simulink library "TQR_lib"  (Simulink 7.5)
settings: Solver=ode45  StartTime=0.0  StopTime=10.0  RelTol=1e-3
values from neighbouring files (symbols this model uses):
  p1_ACPI_PICFilDen1_na = Simulink.Parameter    [TQR_par.m]
  p1_ACPI_PICFilDen2_na = Simulink.Parameter    [TQR_par.m]
  p1_ACPI_PICFilDen3_na = Simulink.Parameter    [TQR_par.m]
  p1_ACPI_PICFilNum1_na = Simulink.Parameter    [TQR_par.m]
  p1_ACPI_PICFilNum2_na = Simulink.Parameter    [TQR_par.m]
  p1_ACPI_PICFilNum3_na = Simulink.Parameter    [TQR_par.m]
  pTQR_bar_BrkPOvrdRecoverThd_C = Simulink.Parameter    [TQR_par.m]
  pTQR_bar_BrkPOvrdVal_C = Simulink.Parameter    [TQR_par.m]
  pTQR_bar_ECrpTrqStrtPres_C = Simulink.Parameter    [TQR_par.m]
  pTQR_bar_MasterCylPres_CUR = Simulink.Parameter    [TQR_par.m]
  pTQR_bool_AccPedOvrdDsbl_C = Simulink.Parameter    [TQR_par.m]
  pTQR_bool_BrkPOvrdDsbl_C = Simulink.Parameter    [TQR_par.m]
  pTQR_bool_BrkRecupSrcSelSwt_C = Simulink.Parameter    [TQR_par.m]
  pTQR_bool_PICTqEna_C = Simulink.Parameter    [TQR_par.m]
  pTQR_bool_RecupEna_C = Simulink.Parameter    [TQR_par.m]
  pTQR_kmph_MaxVehSpd_C = Simulink.Parameter    [TQR_par.m]
  pTQR_kmph_MinVehSpd_C = Simulink.Parameter    [TQR_par.m]
  pTQR_kmph_VehSpd_TAB = Simulink.Parameter    [TQR_par.m]
  pTQR_kmph_VehSpdMaxDriving_TAB = Simulink.Parameter    [TQR_par.m]
  pTQR_kmph_VehSpdMaxReverse_TAB = Simulink.Parameter    [TQR_par.m]
  pTQR_kmph_VehSpdRednHi_CUR = Simulink.Parameter    [TQR_par.m]
  pTQR_kmph_VehSpdRednLo_CUR = Simulink.Parameter    [TQR_par.m]
  pTQR_Nm_ACCDelyOutTrq_C = Simulink.Parameter    [TQR_par.m]
  pTQR_Nm_ACCOutTrqLo_C = Simulink.Parameter    [TQR_par.m]
  pTQR_Nm_ACCOutTrqUp_C = Simulink.Parameter    [TQR_par.m]
  pTQR_Nm_BrkECrpTrq_TAB = Simulink.Parameter    [TQR_par.m]
  pTQR_Nm_MaxRecupTq_C = Simulink.Parameter    [TQR_par.m]
  pTQR_Nm_MotCtlrMaxTqLim_C = Simulink.Parameter    [TQR_par.m]
  pTQR_Nm_MotCtlrMinTqLim_C = Simulink.Parameter    [TQR_par.m]
  pTQR_Nm_PreloadTrq_C = Simulink.Parameter    [TQR_par.m]
  pTQR_Nm_PRNDLoTbl_MAP = Simulink.Parameter    [TQR_par.m]
  pTQR_Nm_RecupLoTbl_MAP = Simulink.Parameter    [TQR_par.m]
  pTQR_Nm_REDEVPRNDLoTbl_MAP = Simulink.Parameter    [TQR_par.m]
  pTQR_Nm_TqLimnUpprLim_C = Simulink.Parameter    [TQR_par.m]
  pTQR_Nmps_AccPedValLowrRateLim_CUR = Simulink.Parameter    [TQR_par.m]
  pTQR_Nmps_AccPedValUpprRateLim_CUR = Simulink.Parameter    [TQR_par.m]
  pTQR_Nmps_CrsCtlLowrRateLim_C = Simulink.Parameter    [TQR_par.m]
  pTQR_Nmps_CrsCtlUpprRateLim_C = Simulink.Parameter    [TQR_par.m]
  pTQR_Nmps_FltLowrRateLim_C = Simulink.Parameter    [TQR_par.m]
  pTQR_Nmps_FltUpprRateLim_C = Simulink.Parameter    [TQR_par.m]
  pTQR_Nmps_LowrRateLimLoTbl_TAB = Simulink.Parameter    [TQR_par.m]
  pTQR_Nmps_UpprRateLimLoTbl_TAB = Simulink.Parameter    [TQR_par.m]
  pTQR_pct_AccPedAcvThd_C = Simulink.Parameter    [TQR_par.m]
  pTQR_pct_AccPedOvrdRecThd_C = Simulink.Parameter    [TQR_par.m]
  pTQR_pct_AccPedOvrdVal_C = Simulink.Parameter    [TQR_par.m]
  pTQR_pct_AccPedThCC_C = Simulink.Parameter    [TQR_par.m]
  pTQR_pct_BrkPOvrdAccPedValThd_C = Simulink.Parameter    [TQR_par.m]
  pTQR_pct_PICAccPedValThd_C = Simulink.Parameter    [TQR_par.m]
  pTQR_r_BrkDwnFilterFac_C = Simulink.Parameter    [TQR_par.m]
  pTQR_r_BrkUpFilterFac_C = Simulink.Parameter    [TQR_par.m]
  pTQR_r_BrkWeightDsbl_C = Simulink.Parameter    [TQR_par.m]
  pTQR_r_BrkWeightFac_C = Simulink.Parameter    [TQR_par.m]
  pTQR_r_ECrpShfFilterFac_C = Simulink.Parameter    [TQR_par.m]
  pTQR_r_PICFilDen1_C = Simulink.Parameter    [TQR_par.m]
  pTQR_r_PICFilDen2_C = Simulink.Parameter    [TQR_par.m]
  pTQR_r_PICFilDen3_C = Simulink.Parameter    [TQR_par.m]
  pTQR_r_PICFilNum1_C = Simulink.Parameter    [TQR_par.m]
  pTQR_r_PICFilNum2_C = Simulink.Parameter    [TQR_par.m]
  pTQR_r_PICFilNum3_C = Simulink.Parameter    [TQR_par.m]
  pTQR_r_PreloadFilterFac_C = Simulink.Parameter    [TQR_par.m]
  pTQR_r_TrqDwnFilterFac_MAP = [ ... (first row only)    [TQR_par.m]
  pTQR_r_TrqUppFilterFac_MAP = [ ... (first row only)    [TQR_par.m]
  pTQR_r_VehSpdFilterFac_CUR = Simulink.Parameter    [TQR_par.m]
  pTQR_ratio_AccPedOvrdLoRate_C = Simulink.Parameter    [TQR_par.m]
  pTQR_ratio_AccPedOvrdUpRate_C = Simulink.Parameter    [TQR_par.m]
  pTQR_ratio_AccPedTqLimUpRate_C = Simulink.Parameter    [TQR_par.m]
  pTQR_ratio_BrkOvrAccPedGrdTh_C = Simulink.Parameter    [TQR_par.m]
  pTQR_ratio_BrkPOvrdLoRate_C = Simulink.Parameter    [TQR_par.m]
  pTQR_ratio_BrkPOvrdUpRate_C = Simulink.Parameter    [TQR_par.m]
  pTQR_ratio_PerfIdxGain_C = Simulink.Parameter    [TQR_par.m]
  pTQR_rpm_VehMoveSpdThrsh_C = Simulink.Parameter    [TQR_par.m]
  pTQR_rpm_VehStdStlSpdThrsh_C = Simulink.Parameter    [TQR_par.m]
  pTQR_s_AccPedActDly_C = Simulink.Parameter    [TQR_par.m]
  pTQR_s_ShfPreloadTrqTmrDly_C = Simulink.Parameter    [TQR_par.m]
  pTQR_s_ShfTrqTmrDly_C = Simulink.Parameter    [TQR_par.m]
  pTQR_s_SmplCyc_C = Simulink.Parameter    [TQR_par.m]
  pTQR_s_VehStdStlDly_C = Simulink.Parameter    [TQR_par.m]
undefined symbols (not defined in the file or in its folder): CrsCtlStsTyp, DiscIntNeverNeededParam, p_single_Minus_M, p_single_Zero_M, ShiftLvrPosnTyp
libraries: BaseOperationLib_Browser x214, simulink x11, PES_CZ_FAW x2, simulink_extras x2, A0EV_Lib1 x1
(part 2 of 2)

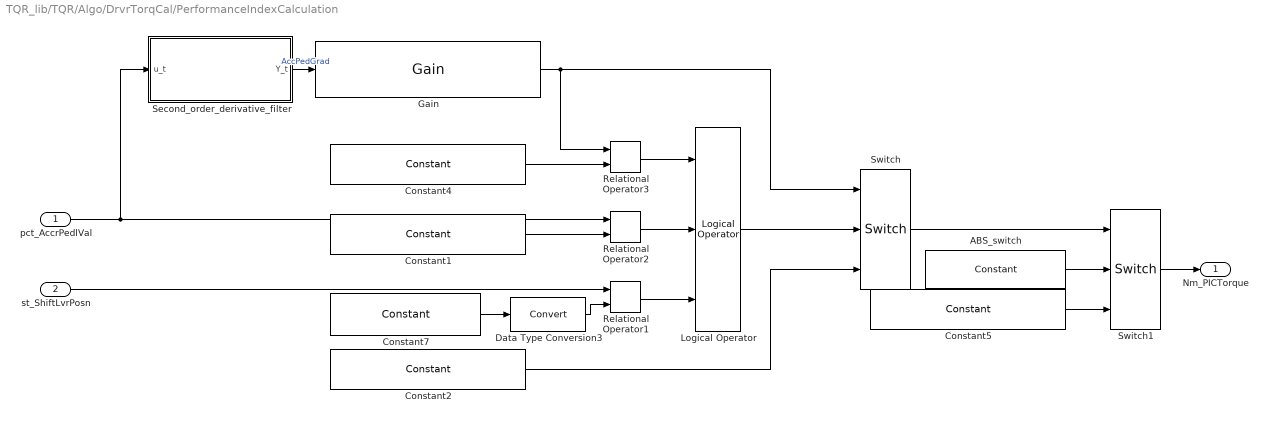
== system TQR_lib/TQR/Algo/DrvrTorqCal/PerformanceIndexCalculation ==
  pct_AccrPedlVal : Inport
  st_ShiftLvrPosn : Inport  Port=2
  ABS_switch : BaseOperationLib_Browser/Sources&Sinks/Constant  Value=pTQR_bool_PICTqEna_C  OutMin=[]  OutMax=[]  OutDataTypeMode=boolean  OutDataType=fixdt(1, 16)  ConRadixGroup=Use specified scaling  OutScaling=2^0  OutDataTypeStr=boolean
  Constant1 : BaseOperationLib_Browser/Sources&Sinks/Constant  Value=pTQR_pct_PICAccPedValThd_C  OutMin=[]  OutMax=[]  OutDataType=fixdt(1, 16)  ConRadixGroup=Use specified scaling  OutScaling=2^0  OutDataTypeStr=Inherit: Inherit from 'Constant value'
  Constant2 : BaseOperationLib_Browser/Sources&Sinks/Constant  Value=p_single_Zero_M  OutMin=[]  OutMax=[]  OutDataType=fixdt(1, 16)  ConRadixGroup=Use specified scaling  OutScaling=2^0  OutDataTypeStr=Inherit: Inherit from 'Constant value'
  Constant4 : BaseOperationLib_Browser/Sources&Sinks/Constant  Value=p_single_Zero_M  OutMin=[]  OutMax=[]  OutDataType=fixdt(1, 16)  ConRadixGroup=Use specified scaling  OutScaling=2^0  OutDataTypeStr=Inherit: Inherit from 'Constant value'
  Constant5 : BaseOperationLib_Browser/Sources&Sinks/Constant  Value=p_single_Zero_M  OutMin=[]  OutMax=[]  OutDataType=fixdt(1, 16)  ConRadixGroup=Use specified scaling  OutScaling=2^0  OutDataTypeStr=Inherit: Inherit from 'Constant value'
  Constant7 : BaseOperationLib_Browser/Sources&Sinks/Constant  Value=ShiftLvrPosnTyp.SHL_D  OutMin=[]  OutMax=[]  OutDataType=fixdt(1, 16)  ConRadixGroup=Use specified scaling  OutScaling=2^0  OutDataTypeStr=Inherit: Inherit from 'Constant value'
  Data Type Conversion3 : DataTypeConversion  OutDataType=fixdt(1, 16)  OutScaling=2^0
  Gain : BaseOperationLib_Browser/Math Operations Changed/Gain  Gain=pTQR_ratio_PerfIdxGain_C  Multiplication=Element-wise(K.*u)  ParamMin=[]  ParamMax=[]  ParameterDataType=fixdt(1, 16)  ParameterScalingMode=Best Precision: Matrix-wise  ParameterScaling=2^0  OutMin=[]  OutMax=[]  OutDataType=fixdt(1, 16)  OutScaling=2^0  OutDataTypeStr=Inherit: Inherit via back propagation
  Logical Operator : BaseOperationLib_Browser/Logic Operations Changed/Logical Operator  Operator=AND  Inputs=3  AllPortsSameDT=off  OutDataTypeMode=boolean  LogicDataType=PDT_Bool  OutDataTypeStr=boolean
  Relational Operator1 : BaseOperationLib_Browser/Logic Operations Changed/Relational Operator  Operator===  LogicOutDataTypeMode=boolean  LogicDataType=PDT_Bool  OutDataTypeStr=boolean
  Relational Operator2 : BaseOperationLib_Browser/Logic Operations Changed/Relational Operator  Operator=>  LogicOutDataTypeMode=boolean  LogicDataType=PDT_Bool  OutDataTypeStr=boolean
  Relational Operator3 : BaseOperationLib_Browser/Logic Operations Changed/Relational Operator  Operator=>  LogicOutDataTypeMode=boolean  LogicDataType=PDT_Bool  OutDataTypeStr=boolean
  Second_order_derivative_filter : Subsystem
  Switch : BaseOperationLib_Browser/Signal Routing Changed/Switch  Criteria=u2 ~= 0  Threshold=0  OutMin=[]  OutMax=[]  OutDataType=fixdt(1,16,0)  OutScaling=[]
  Switch1 : BaseOperationLib_Browser/Signal Routing Changed/Switch  Criteria=u2 ~= 0  Threshold=0  OutMin=[]  OutMax=[]  OutDataType=fixdt(1,16,0)  OutScaling=[]
  Nm_PICTorque : Outport
  wires:
  Gain/1 -> Switch/1, Relational Operator3/1
  Constant2/1 -> Switch/3
  Logical Operator/1 -> Switch/2
  pct_AccrPedlVal/1 -> Relational Operator2/1, Second_order_derivative_filter/1(u_t)
  Constant1/1 -> Relational Operator2/2
  Second_order_derivative_filter/1(Y_t) -> Gain/1  "AccPedGrad"
  Relational Operator3/1 -> Logical Operator/1
  Constant4/1 -> Relational Operator3/2
  Relational Operator2/1 -> Logical Operator/2
  Switch/1 -> Switch1/1
  Constant5/1 -> Switch1/3
  ABS_switch/1 -> Switch1/2
  Switch1/1 -> Nm_PICTorque/1
  Data Type Conversion3/1 -> Relational Operator1/2
  Constant7/1 -> Data Type Conversion3/1
  Relational Operator1/1 -> Logical Operator/3
  st_ShiftLvrPosn/1 -> Relational Operator1/1

== system TQR_lib/TQR/Algo/DrvrTorqCal/SlpVehLgtSpdTrans ==
  kmph_VehLgtSpd : Inport
  st_ShiftLvrPosn : Inport  Port=2
  Constant1 : BaseOperationLib_Browser/Sources&Sinks/Constant  Value=pTQR_kmph_MaxVehSpd_C  OutMin=[]  OutMax=[]  OutDataType=fixdt(1, 16)  ConRadixGroup=Use specified scaling  OutScaling=2^0  OutDataTypeStr=Inherit: Inherit from 'Constant value'
  Constant3 : BaseOperationLib_Browser/Sources&Sinks/Constant  Value=pTQR_kmph_MinVehSpd_C  OutMin=[]  OutMax=[]  OutDataType=fixdt(1, 16)  ConRadixGroup=Use specified scaling  OutScaling=2^0  OutDataTypeStr=Inherit: Inherit from 'Constant value'
  Constant7 : BaseOperationLib_Browser/Sources&Sinks/Constant  Value=ShiftLvrPosnTyp.SHL_R  OutMin=[]  OutMax=[]  OutDataType=fixdt(1, 16)  ConRadixGroup=Use specified scaling  OutScaling=2^0  OutDataTypeStr=Inherit: Inherit from 'Constant value'
  Data Type Conversion3 : DataTypeConversion  OutDataType=fixdt(1, 16)  OutScaling=2^0
  ECrpVehSpdFilter : Subsystem
  Gain : BaseOperationLib_Browser/Math Operations Changed/Gain  Gain=p_single_Minus_M  Multiplication=Element-wise(K.*u)  ParamMin=[]  ParamMax=[]  ParameterDataType=fixdt(1, 16)  ParameterScalingMode=Best Precision: Matrix-wise  ParameterScaling=2^0  ParamDataTypeStr=Inherit: Inherit from 'Gain'  OutMin=[]  OutMax=[]  OutDataType=fixdt(1, 16)  OutScaling=2^0  SaturateOnIntegerOverflow=on
  Relational Operator1 : BaseOperationLib_Browser/Logic Operations Changed/Relational Operator  Operator===  LogicOutDataTypeMode=boolean  LogicDataType=PDT_Bool  OutDataTypeStr=boolean
  Saturation Dynamic : BaseOperationLib_Browser/Discontinuities Unchanged/Saturation Dynamic  SystemSampleTime=-1  OutMin=[]  OutMax=[]  OutDataTypeStr=Inherit: Same as second input  OutDataType=fixdt(1, 16)  OutScaling=2^-10  DoSatur=off
  Switch2 : BaseOperationLib_Browser/Signal Routing Changed/Switch  Criteria=u2 ~= 0  Threshold=0  OutMin=[]  OutMax=[]  OutDataType=fixdt(1,16,0)  OutScaling=[]
  kmph_SlpVehLgtSpdTrans : Outport
  wires:
  Data Type Conversion3/1 -> Relational Operator1/2
  Constant7/1 -> Data Type Conversion3/1
  Relational Operator1/1 -> Switch2/2
  kmph_VehLgtSpd/1 -> Switch2/3, Gain/1
  st_ShiftLvrPosn/1 -> Relational Operator1/1
  Constant3/1 -> Saturation Dynamic/3
  Constant1/1 -> Saturation Dynamic/1
  Switch2/1 -> Saturation Dynamic/2
  ECrpVehSpdFilter/1(kmph_VehSpdFilter) -> kmph_SlpVehLgtSpdTrans/1
  Saturation Dynamic/1 -> ECrpVehSpdFilter/1(kmph_VehSpd)
  Gain/1 -> Switch2/1

== system TQR_lib/TQR/Algo/DrvrTorqCal/velocity_limitation ==
  Nm_MotCtlrTqSp : Inport
  st_ShiftLvrPosn : Inport  Port=2
  kmph_VehLgtSpd : Inport  Port=3
  1-D Lookup Table_TQ_D : Lookup_n-D  NumberOfTableDimensions=1  BreakpointsForDimension1=pTQR_kmph_VehSpdMaxDriving_TAB  Table=[1 1 0 0]  RndMeth=Simplest  InputSameDT=on
  1-D Lookup Table_TQ_R : Lookup_n-D  NumberOfTableDimensions=1  BreakpointsForDimension1=pTQR_kmph_VehSpdMaxReverse_TAB  Table=[1 1 0 0]  RndMeth=Simplest  InputSameDT=on
  Abs : BaseOperationLib_Browser/Math Operations Changed/Abs  OutMax=[]  OutDataType=fixdt(1, 16)  OutScaling=2^0
  Compare To Zero : simulink/Logic and Bit Operations/Compare To Zero  SystemSampleTime=-1  relop=>  LogicOutDataTypeMode=uint8
  Constant : BaseOperationLib_Browser/Sources&Sinks/Constant  Value=ShiftLvrPosnTyp.SHL_R  OutMin=[]  OutMax=[]  OutDataTypeMode=Specify via dialog  OutDataType=Enum: ShiftLvrPosnTyp  ConRadixGroup=Best Precision: Vector-wise  OutScaling=[]  OutDataTypeStr=Enum: ShiftLvrPosnTyp
  Data Type Conversion1 : DataTypeConversion  OutDataType=fixdt(1, 16)  OutScaling=2^0
  Data Type Conversion2 : DataTypeConversion  OutDataTypeMode=Specify via dialog  OutDataType=Enum: ShiftLvrPosnTyp  OutDataTypeStr=Enum: ShiftLvrPosnTyp
  Product1 : BaseOperationLib_Browser/Math Operations Changed/Product  Inputs=2  Multiplication=Element-wise(.*)  OutMin=[]  OutMax=[]  OutDataType=fixdt(1,16,0)  OutScaling=[]  RndMeth=Zero
  Relational Operator : BaseOperationLib_Browser/Logic Operations Changed/Relational Operator  Operator===  LogicOutDataTypeMode=boolean  LogicDataType=PDT_Bool  OutDataTypeStr=boolean
  Switch : BaseOperationLib_Browser/Signal Routing Changed/Switch  Criteria=u2 ~= 0  Threshold=0  OutMin=[]  OutMax=[]  OutDataType=fixdt(1,16,0)  OutScaling=[]
  Switch1 : BaseOperationLib_Browser/Signal Routing Changed/Switch  Criteria=u2 ~= 0  Threshold=0  OutMin=[]  OutMax=[]  OutDataType=fixdt(1,16,0)  OutScaling=[]
  Nm_SpdLimitMotCtlrTqSp : Outport
  wires:
  Switch1/1 -> Data Type Conversion1/1
  Product1/1 -> Switch1/1
  Compare To Zero/1 -> Switch1/2
  Data Type Conversion2/1 -> Relational Operator/1
  Constant/1 -> Relational Operator/2
  Relational Operator/1 -> Switch/2
  1-D Lookup Table_TQ_D/1 -> Switch/3
  1-D Lookup Table_TQ_R/1 -> Switch/1
  Switch/1 -> Product1/1
  st_ShiftLvrPosn/1 -> Data Type Conversion2/1
  Nm_MotCtlrTqSp/1 -> Switch1/3, Product1/2, Compare To Zero/1
  kmph_VehLgtSpd/1 -> Abs/1
  Data Type Conversion1/1 -> Nm_SpdLimitMotCtlrTqSp/1
  Abs/1 -> 1-D Lookup Table_TQ_D/1, 1-D Lookup Table_TQ_R/1

== system TQR_lib/TQR/Algo/TorqArbitrition/DriveTorqArbitrition ==
  pct_AccrPedlVal : Inport
  Nm_CrsCtlTqSp : Inport  Port=2
  st_CrsCtlEna : Inport  Port=3
  Nm_TorqueRaw : Inport  Port=4
  Compare To Constant1 : BaseOperationLib_Browser/Logic Operations Changed/Compare To Constant  SystemSampleTime=-1  relop=>=  const=pTQR_pct_AccPedThCC_C
  Constant1 : BaseOperationLib_Browser/Sources&Sinks/Constant  Value=uint8(CrsCtlStsTyp.CCS_ACTIVE)  OutMin=[]  OutMax=[]  OutDataType=fixdt(1, 16)  ConRadixGroup=Use specified scaling  OutScaling=2^0  OutDataTypeStr=Inherit: Inherit from 'Constant value'
  Logical Operator : BaseOperationLib_Browser/Logic Operations Changed/Logical Operator  Operator=AND  Inputs=2  AllPortsSameDT=off  OutDataTypeMode=boolean  LogicDataType=PDT_Bool  OutDataTypeStr=boolean
  Logical Operator4 : BaseOperationLib_Browser/Logic Operations Changed/Logical Operator  Operator=NOT  Inputs=3  AllPortsSameDT=off  OutDataTypeMode=boolean  LogicDataType=PDT_Bool  OutDataTypeStr=boolean
  Logical Operator5 : BaseOperationLib_Browser/Logic Operations Changed/Logical Operator  Operator=OR  Inputs=2  AllPortsSameDT=off  OutDataTypeMode=boolean  LogicDataType=PDT_Bool  OutDataTypeStr=boolean
  MinMax : BaseOperationLib_Browser/Math Operations Changed/MinMax  Function=max  Inputs=2  OutMin=[]  OutMax=[]  OutDataType=fixdt(1, 16)  OutScaling=2^0
  Relational Operator : BaseOperationLib_Browser/Logic Operations Changed/Relational Operator  Operator=>=  LogicOutDataTypeMode=boolean  LogicDataType=PDT_Bool  OutDataTypeStr=boolean
  Relational Operator2 : BaseOperationLib_Browser/Logic Operations Changed/Relational Operator  Operator===  LogicOutDataTypeMode=boolean  LogicDataType=PDT_Bool  OutDataTypeStr=boolean
  Switch1 : BaseOperationLib_Browser/Signal Routing Changed/Switch  Criteria=u2 ~= 0  Threshold=0  OutMin=[]  OutMax=[]  OutDataType=fixdt(1,16,0)  OutScaling=[]
  Switch2 : BaseOperationLib_Browser/Signal Routing Changed/Switch  Criteria=u2 ~= 0  Threshold=0  OutMin=[]  OutMax=[]  OutDataType=fixdt(1,16,0)  OutScaling=[]
  Nm_DriveTorq : Outport
  bool_CrsCtlActive : Outport  Port=2
  wires:
  Constant1/1 -> Relational Operator2/1
  Switch2/1 -> Switch1/1
  MinMax/1 -> Switch2/1
  Compare To Constant1/1 -> Switch2/2, Logical Operator4/1
  Nm_TorqueRaw/1 -> MinMax/2, Switch1/3, Relational Operator/2
  Nm_CrsCtlTqSp/1 -> Switch2/3, MinMax/1, Relational Operator/1
  Relational Operator/1 -> Logical Operator5/2
  Logical Operator4/1 -> Logical Operator5/1
  Logical Operator5/1 -> Logical Operator/1
  Relational Operator2/1 -> Switch1/2, Logical Operator/2
  pct_AccrPedlVal/1 -> Compare To Constant1/1
  Switch1/1 -> Nm_DriveTorq/1
  st_CrsCtlEna/1 -> Relational Operator2/2
  Logical Operator/1 -> bool_CrsCtlActive/1

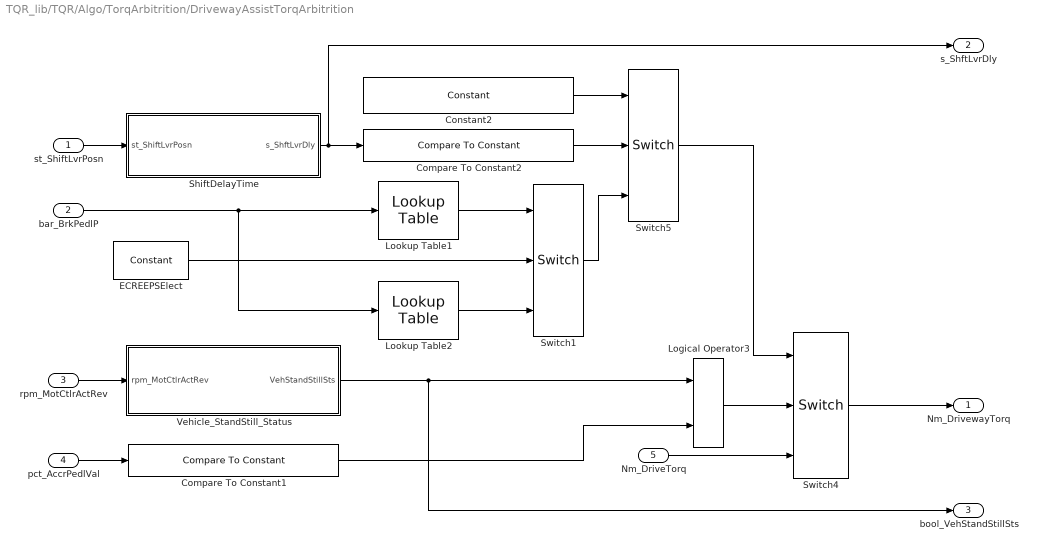
== system TQR_lib/TQR/Algo/TorqArbitrition/DrivewayAssistTorqArbitrition ==
  st_ShiftLvrPosn : Inport
  bar_BrkPedlP : Inport  Port=2
  rpm_MotCtlrActRev : Inport  Port=3
  pct_AccrPedlVal : Inport  Port=4
  Nm_DriveTorq : Inport  Port=5
  Compare To Constant1 : BaseOperationLib_Browser/Logic Operations Changed/Compare To Constant  SystemSampleTime=-1  relop=<  const=pTQR_pct_AccPedThCC_C
  Compare To Constant2 : BaseOperationLib_Browser/Logic Operations Changed/Compare To Constant  SystemSampleTime=-1  relop=<=  const=pTQR_s_ShfPreloadTrqTmrDly_C
  Constant2 : BaseOperationLib_Browser/Sources&Sinks/Constant  Value=pTQR_Nm_PreloadTrq_C  OutMin=[]  OutMax=[]  OutDataType=fixdt(1, 16)  ConRadixGroup=Use specified scaling  OutScaling=2^0  OutDataTypeStr=Inherit: Inherit from 'Constant value'
  ECREEPSElect : BaseOperationLib_Browser/Sources&Sinks/Constant  Value=0  OutMin=[]  OutMax=[]  OutDataType=fixdt(1, 16)  ConRadixGroup=Use specified scaling  OutScaling=2^0  OutDataTypeStr=Inherit: Inherit from 'Constant value'
  Logical Operator3 : BaseOperationLib_Browser/Logic Operations Changed/Logical Operator  Operator=AND  Inputs=2  AllPortsSameDT=off  OutDataTypeMode=boolean  LogicDataType=PDT_Bool  OutDataTypeStr=boolean
  Lookup Table1 : BaseOperationLib_Browser/Lookup Tables Changed/Lookup Table  InputValues=pTQR_bar_MasterCylPres_CUR  Table=pTQR_Nm_BrkECrpTrq_TAB  LookUpMeth=Interpolation-Use End Values  OutMin=[]  OutMax=[]  OutDataType=fixdt(1, 16)  OutScaling=2^0  OutDataTypeStr=Inherit: Inherit via back propagation  SaturateOnIntegerOverflow=on
      settings: AttributesFormatString=X:%<InputValues>\nTAB:%<Table>
  Lookup Table2 : BaseOperationLib_Browser/Lookup Tables Changed/Lookup Table  InputValues=[0 4.4 4.6 5 200]  Table=[60 60 4 0 0]  LookUpMeth=Interpolation-Use End Values  OutMin=[]  OutMax=[]  OutDataType=fixdt(1, 16)  OutScaling=2^0  OutDataTypeStr=Inherit: Inherit via back propagation  SaturateOnIntegerOverflow=on
      settings: AttributesFormatString=X:%<InputValues>\nTAB:%<Table>
  ShiftDelayTime : Subsystem
  Switch1 : BaseOperationLib_Browser/Signal Routing Changed/Switch  Criteria=u2 ~= 0  Threshold=0  OutMin=[]  OutMax=[]  OutDataType=fixdt(1,16,0)  OutScaling=[]
  Switch4 : BaseOperationLib_Browser/Signal Routing Changed/Switch  Criteria=u2 ~= 0  Threshold=0  OutMin=[]  OutMax=[]  OutDataType=fixdt(1,16,0)  OutScaling=[]
  Switch5 : BaseOperationLib_Browser/Signal Routing Changed/Switch  Criteria=u2 ~= 0  Threshold=0  OutMin=[]  OutMax=[]  OutDataType=fixdt(1,16,0)  OutScaling=[]
  Vehicle_StandStill_Status : Subsystem
  Nm_DrivewayTorq : Outport
  s_ShftLvrDly : Outport  Port=2  PortDimensions=1  OutDataType=fixdt(1, 16)  OutScaling=2^0
  bool_VehStandStillSts : Outport  Port=3
  wires:
  ECREEPSElect/1 -> Switch1/2
  Switch1/1 -> Switch5/3
  Lookup Table1/1 -> Switch1/1
  Lookup Table2/1 -> Switch1/3
  ShiftDelayTime/1(s_ShftLvrDly) -> Compare To Constant2/1, s_ShftLvrDly/1
  rpm_MotCtlrActRev/1 -> Vehicle_StandStill_Status/1(rpm_MotCtlrActRev)
  Vehicle_StandStill_Status/1(VehStandStillSts) -> Logical Operator3/1, bool_VehStandStillSts/1
  bar_BrkPedlP/1 -> Lookup Table1/1, Lookup Table2/1
  Logical Operator3/1 -> Switch4/2
  Compare To Constant1/1 -> Logical Operator3/2
  Switch5/1 -> Switch4/1
  Constant2/1 -> Switch5/1
  Compare To Constant2/1 -> Switch5/2
  st_ShiftLvrPosn/1 -> ShiftDelayTime/1(st_ShiftLvrPosn)
  Switch4/1 -> Nm_DrivewayTorq/1
  Nm_DriveTorq/1 -> Switch4/3
  pct_AccrPedlVal/1 -> Compare To Constant1/1

== system TQR_lib/TQR/Algo/TorqueLimit/no_recuperation ==
  Nm_ReductionTorq : Inport
  React_Bus : Inport  Port=2
  Constant2 : BaseOperationLib_Browser/Sources&Sinks/Constant  Value=p_single_Zero_M  OutMin=[]  OutMax=[]  OutDataTypeMode=single  OutDataType=fixdt(1, 16)  ConRadixGroup=Use specified scaling  OutScaling=2^0  OutDataTypeStr=single
  GetBit1 : Subsystem  mask{maska=FtlReactDTRTyp.NO_RECUPERATION}
      mask prompts: maska "bitAND with parameter"
      mask help:
      | Get Bit
      |
      | Implements Masked AND between the input and mask. If the result is grater than zero true is set to output - otherwise false.
      |
      | Block is useful for decoding bit-encoded data.
      |
      | Mask may not be a calibratable parameter.
      mask Help:
      | Get Bit
      | 
      | Implements Masked AND between the input and mask. If the result is grater than zero true is set to output - otherwise false.
      | 
      | Block is useful for decoding bit-encoded data.
      | 
      | Mask may not be a calibratable parameter.
      mask Display: disp(['Input bitAND \n',maska]);
  Logical Operator3 : BaseOperationLib_Browser/Logic Operations Changed/Logical Operator  Operator=NOT  Inputs=2  AllPortsSameDT=off  OutDataTypeMode=boolean  LogicDataType=PDT_Bool  OutDataTypeStr=boolean
  Logical Operator4 : BaseOperationLib_Browser/Logic Operations Changed/Logical Operator  Operator=AND  Inputs=2  AllPortsSameDT=off  OutDataTypeMode=boolean  LogicDataType=PDT_Bool  OutDataTypeStr=boolean
  MinMax1 : BaseOperationLib_Browser/Math Operations Changed/MinMax  Function=max  Inputs=2  InputSameDT=on  OutMin=[]  OutMax=[]  OutDataType=fixdt(1, 16)  OutScaling=2^0  SaturateOnIntegerOverflow=on
  Recup_enable : BaseOperationLib_Browser/Sources&Sinks/Constant  Value=pTQR_bool_RecupEna_C  OutMin=[]  OutMax=[]  OutDataTypeMode=boolean  OutDataType=fixdt(1, 16)  ConRadixGroup=Use specified scaling  OutScaling=2^0  OutDataTypeStr=boolean
  Switch : BaseOperationLib_Browser/Signal Routing Changed/Switch  Criteria=u2 ~= 0  Threshold=0  OutMin=[]  OutMax=[]  OutDataType=fixdt(1,16,0)  OutScaling=[]
  Nm_NoRecupTorq : Outport
  wires:
  Logical Operator3/1 -> Logical Operator4/2
  Recup_enable/1 -> Logical Operator4/1
  Logical Operator4/1 -> Switch/2
  GetBit1/1(Out1) -> Logical Operator3/1
  React_Bus/1 -> GetBit1/1(In1)
  Nm_ReductionTorq/1 -> Switch/1, MinMax1/1
  Switch/1 -> Nm_NoRecupTorq/1
  MinMax1/1 -> Switch/3
  Constant2/1 -> MinMax1/2

== system TQR_lib/TQR/Algo/TorqueLimit/torque_reduction ==
  Nm_VelReducTorq : Inport
  React_Bus : Inport  Port=2
  Constant : BaseOperationLib_Browser/Sources&Sinks/Constant  Value=pTQR_Nm_MotCtlrMaxTqLim_C  OutMin=[]  OutMax=[]  OutDataType=fixdt(1, 16)  ConRadixGroup=Use specified scaling  OutScaling=2^0  OutDataTypeStr=Inherit: Inherit from 'Constant value'
  Constant1 : BaseOperationLib_Browser/Sources&Sinks/Constant  Value=pTQR_Nm_MotCtlrMinTqLim_C  OutMin=[]  OutMax=[]  OutDataType=fixdt(1, 16)  ConRadixGroup=Use specified scaling  OutScaling=2^0  OutDataTypeStr=Inherit: Inherit from 'Constant value'
  GetBit2 : Subsystem  mask{maska=FtlReactDTRTyp.TORQUE_REDUCTION}
      mask prompts: maska "bitAND with parameter"
      mask help:
      | Get Bit
      |
      | Implements Masked AND between the input and mask. If the result is grater than zero true is set to output - otherwise false.
      |
      | Block is useful for decoding bit-encoded data.
      |
      | Mask may not be a calibratable parameter.
      mask Help:
      | Get Bit
      | 
      | Implements Masked AND between the input and mask. If the result is grater than zero true is set to output - otherwise false.
      | 
      | Block is useful for decoding bit-encoded data.
      | 
      | Mask may not be a calibratable parameter.
      mask Display: disp(['Input bitAND \n',maska]);
  Saturation Dynamic : BaseOperationLib_Browser/Discontinuities Unchanged/Saturation Dynamic  SystemSampleTime=-1  OutMin=[]  OutMax=[]  OutDataTypeStr=Inherit: Same as second input  OutDataType=fixdt(1, 16)  OutScaling=2^-10  DoSatur=off
  Switch2 : BaseOperationLib_Browser/Signal Routing Changed/Switch  Criteria=u2 ~= 0  Threshold=0  OutMin=[]  OutMax=[]  OutDataType=fixdt(1,16,0)  OutScaling=[]
  Nm_ReductionTorq : Outport
  wires:
  GetBit2/1(Out1) -> Switch2/2
  Constant/1 -> Saturation Dynamic/1
  Constant1/1 -> Saturation Dynamic/3
  Saturation Dynamic/1 -> Switch2/1
  Nm_VelReducTorq/1 -> Switch2/3, Saturation Dynamic/2
  React_Bus/1 -> GetBit2/1(In1)
  Switch2/1 -> Nm_ReductionTorq/1

== system TQR_lib/TQR/Algo/TorqueLimit/velocity_reduction ==
  Nm_MotCtlrTqSp : Inport
  kmph_VehLgtSpd : Inport  Port=2
  React_Bus : Inport  Port=3
  1-D Lookup Table_TQ_Reduction_HIGH : Lookup_n-D  NumberOfTableDimensions=1  BreakpointsForDimension1=pTQR_kmph_VehSpdRednHi_CUR  Table=[1 1 0 0]  RndMeth=Simplest  InputSameDT=on
  1-D Lookup Table_TQ_Reduction_LOW : Lookup_n-D  NumberOfTableDimensions=1  BreakpointsForDimension1=pTQR_kmph_VehSpdRednLo_CUR  Table=[1 1 0 0]  RndMeth=Simplest  InputSameDT=on
  Abs : BaseOperationLib_Browser/Math Operations Changed/Abs  OutMax=[]  OutDataType=fixdt(1, 16)  OutScaling=2^0
  Compare To Zero : simulink/Logic and Bit Operations/Compare To Zero  SystemSampleTime=-1  relop=>  LogicOutDataTypeMode=uint8
  GetBit1 : Subsystem  mask{maska=FtlReactDTRTyp.VELOCITY_REDUCTION_HIGH}
      mask prompts: maska "bitAND with parameter"
      mask help:
      | Get Bit
      |
      | Implements Masked AND between the input and mask. If the result is grater than zero true is set to output - otherwise false.
      |
      | Block is useful for decoding bit-encoded data.
      |
      | Mask may not be a calibratable parameter.
      mask Help:
      | Get Bit
      | 
      | Implements Masked AND between the input and mask. If the result is grater than zero true is set to output - otherwise false.
      | 
      | Block is useful for decoding bit-encoded data.
      | 
      | Mask may not be a calibratable parameter.
      mask Display: disp(['Input bitAND \n',maska]);
  GetBit2 : Subsystem  mask{maska=FtlReactDTRTyp.VELOCITY_REDUCTION_LOW}
      mask prompts: maska "bitAND with parameter"
      mask help:
      | Get Bit
      |
      | Implements Masked AND between the input and mask. If the result is grater than zero true is set to output - otherwise false.
      |
      | Block is useful for decoding bit-encoded data.
      |
      | Mask may not be a calibratable parameter.
      mask Help:
      | Get Bit
      | 
      | Implements Masked AND between the input and mask. If the result is grater than zero true is set to output - otherwise false.
      | 
      | Block is useful for decoding bit-encoded data.
      | 
      | Mask may not be a calibratable parameter.
      mask Display: disp(['Input bitAND \n',maska]);
  Logical Operator : BaseOperationLib_Browser/Logic Operations Changed/Logical Operator  Operator=OR  Inputs=2  AllPortsSameDT=off  OutDataTypeMode=boolean  LogicDataType=PDT_Bool  OutDataTypeStr=boolean
  Product1 : BaseOperationLib_Browser/Math Operations Changed/Product  Inputs=2  Multiplication=Element-wise(.*)  OutMin=[]  OutMax=[]  OutDataType=fixdt(1,16,0)  OutScaling=[]  RndMeth=Zero
  Switch : BaseOperationLib_Browser/Signal Routing Changed/Switch  Criteria=u2 ~= 0  Threshold=0  OutMin=[]  OutMax=[]  OutDataType=fixdt(1,16,0)  OutScaling=[]
  Switch4 : BaseOperationLib_Browser/Signal Routing Changed/Switch  Criteria=u2 ~= 0  Threshold=0  OutMin=[]  OutMax=[]  OutDataType=fixdt(1,16,0)  OutScaling=[]
  Switch5 : BaseOperationLib_Browser/Signal Routing Changed/Switch  Criteria=u2 ~= 0  Threshold=0  OutMin=[]  OutMax=[]  OutDataType=fixdt(1,16,0)  OutScaling=[]
  Nm_VelReducTrq : Outport
  wires:
  Switch5/1 -> Switch/1
  Compare To Zero/1 -> Switch5/2
  Switch4/1 -> Product1/2
  1-D Lookup Table_TQ_Reduction_HIGH/1 -> Switch4/3
  1-D Lookup Table_TQ_Reduction_LOW/1 -> Switch4/1
  Logical Operator/1 -> Switch/2
  GetBit1/1(Out1) -> Logical Operator/2
  GetBit2/1(Out1) -> Switch4/2, Logical Operator/1
  Product1/1 -> Switch5/1
  Abs/1 -> 1-D Lookup Table_TQ_Reduction_HIGH/1, 1-D Lookup Table_TQ_Reduction_LOW/1
  React_Bus/1 -> GetBit2/1(In1), GetBit1/1(In1)
  kmph_VehLgtSpd/1 -> Abs/1
  Switch/1 -> Nm_VelReducTrq/1
  Nm_MotCtlrTqSp/1 -> Compare To Zero/1, Switch5/3, Switch/3, Product1/1

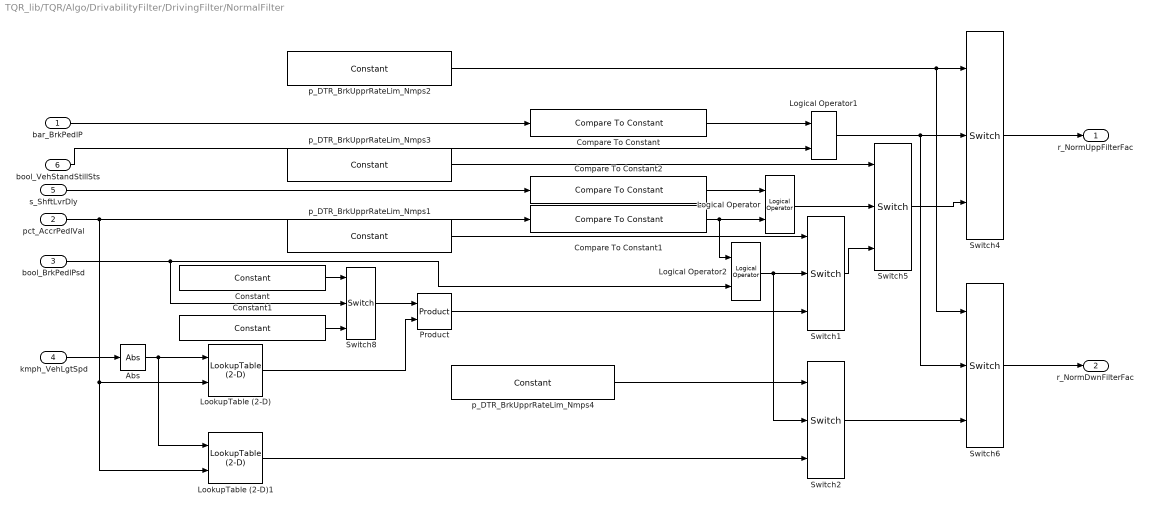
== system TQR_lib/TQR/Algo/DrivabilityFilter/DrivingFilter/NormalFilter ==
  bar_BrkPedlP : Inport
  pct_AccrPedlVal : Inport  Port=2
  bool_BrkPedlPsd : Inport  Port=3
  kmph_VehLgtSpd : Inport  Port=4
  s_ShftLvrDly : Inport  Port=5
  bool_VehStandStillSts : Inport  Port=6
  Abs : BaseOperationLib_Browser/Math Operations Changed/Abs  OutMax=[]  OutDataType=fixdt(1, 16)  OutScaling=2^0
  Compare To Constant : BaseOperationLib_Browser/Logic Operations Changed/Compare To Constant  SystemSampleTime=-1  relop=>=  const=pTQR_bar_ECrpTrqStrtPres_C
  Compare To Constant1 : BaseOperationLib_Browser/Logic Operations Changed/Compare To Constant  SystemSampleTime=-1  relop=<=  const=pTQR_pct_AccPedAcvThd_C
  Compare To Constant2 : BaseOperationLib_Browser/Logic Operations Changed/Compare To Constant  SystemSampleTime=-1  relop=<=  const=pTQR_s_ShfTrqTmrDly_C
  Constant : BaseOperationLib_Browser/Sources&Sinks/Constant  Value=pTQR_r_BrkWeightFac_C  OutMin=[]  OutMax=[]  OutDataType=fixdt(1, 16)  ConRadixGroup=Use specified scaling  OutScaling=2^0  OutDataTypeStr=Inherit: Inherit from 'Constant value'
  Constant1 : BaseOperationLib_Browser/Sources&Sinks/Constant  Value=pTQR_r_BrkWeightDsbl_C  OutMin=[]  OutMax=[]  OutDataType=fixdt(1, 16)  ConRadixGroup=Use specified scaling  OutScaling=2^0  OutDataTypeStr=Inherit: Inherit from 'Constant value'
  Logical Operator : BaseOperationLib_Browser/Logic Operations Changed/Logical Operator  Operator=AND  Inputs=2  AllPortsSameDT=off  OutDataTypeMode=boolean  LogicDataType=PDT_Bool  OutDataTypeStr=boolean
  Logical Operator1 : BaseOperationLib_Browser/Logic Operations Changed/Logical Operator  Operator=AND  Inputs=2  AllPortsSameDT=off  OutDataTypeMode=boolean  LogicDataType=PDT_Bool  OutDataTypeStr=boolean
  Logical Operator2 : BaseOperationLib_Browser/Logic Operations Changed/Logical Operator  Operator=AND  Inputs=2  AllPortsSameDT=off  OutDataTypeMode=boolean  LogicDataType=PDT_Bool  OutDataTypeStr=boolean
  LookupTable (2-D) : BaseOperationLib_Browser/Lookup Tables Changed/LookupTable (2-D)  RowIndex=pTQR_kmph_TrqFilterVsp_TABX  ColumnIndex=pTQR_pct_TrqFilterAccPed_TABY  Table=pTQR_r_TrqUppFilterFac_MAP  LookUpMeth=Interpolation-Use End Values  OutMin=[]  OutMax=[]  OutDataType=fixdt(1, 16)  OutScaling=2^0  OutDataTypeStr=Inherit: Inherit via back propagation  SaturateOnIntegerOverflow=on
      settings: AttributesFormatString=X:%<RowIndex>\nY:%<ColumnIndex>\nTAB:%<Table>
  LookupTable (2-D)1 : BaseOperationLib_Browser/Lookup Tables Changed/LookupTable (2-D)  RowIndex=pTQR_kmph_TrqFilterVsp_TABX  ColumnIndex=pTQR_pct_TrqFilterAccPed_TABY  Table=pTQR_r_TrqDwnFilterFac_MAP  LookUpMeth=Interpolation-Use End Values  OutMin=[]  OutMax=[]  OutDataType=fixdt(1, 16)  OutScaling=2^0  OutDataTypeStr=Inherit: Inherit via back propagation  SaturateOnIntegerOverflow=on
      settings: AttributesFormatString=X:%<RowIndex>\nY:%<ColumnIndex>\nTAB:%<Table>
  Product : BaseOperationLib_Browser/Math Operations Changed/Product  Inputs=2  Multiplication=Element-wise(.*)  OutMin=[]  OutMax=[]  OutDataType=fixdt(1,16,0)  OutScaling=[]  OutDataTypeStr=Inherit: Inherit via back propagation  RndMeth=Zero  SaturateOnIntegerOverflow=on
  Switch{1..2,4..6,8} (6 alike) : BaseOperationLib_Browser/Signal Routing Changed/Switch  Criteria=u2 ~= 0  Threshold=0  OutMin=[]  OutMax=[]  OutDataType=fixdt(1,16,0)  OutScaling=[]
  p_DTR_BrkUpprRateLim_Nmps1 : BaseOperationLib_Browser/Sources&Sinks/Constant  Value=pTQR_r_BrkUpFilterFac_C  OutMin=[]  OutMax=[]  OutDataTypeMode=single  OutDataType=fixdt(1, 16)  ConRadixGroup=Use specified scaling  OutScaling=2^0  OutDataTypeStr=single
  p_DTR_BrkUpprRateLim_Nmps2 : BaseOperationLib_Browser/Sources&Sinks/Constant  Value=pTQR_r_PreloadFilterFac_C  OutMin=[]  OutMax=[]  OutDataTypeMode=single  OutDataType=fixdt(1, 16)  ConRadixGroup=Use specified scaling  OutScaling=2^0  OutDataTypeStr=single
  p_DTR_BrkUpprRateLim_Nmps3 : BaseOperationLib_Browser/Sources&Sinks/Constant  Value=pTQR_r_ECrpShfFilterFac_C  OutMin=[]  OutMax=[]  OutDataTypeMode=single  OutDataType=fixdt(1, 16)  ConRadixGroup=Use specified scaling  OutScaling=2^0  OutDataTypeStr=single
  p_DTR_BrkUpprRateLim_Nmps4 : BaseOperationLib_Browser/Sources&Sinks/Constant  Value=pTQR_r_BrkDwnFilterFac_C  OutMin=[]  OutMax=[]  OutDataTypeMode=single  OutDataType=fixdt(1, 16)  ConRadixGroup=Use specified scaling  OutScaling=2^0  OutDataTypeStr=single
  r_NormUppFilterFac : Outport
  r_NormDwnFilterFac : Outport  Port=2
  wires:
  Switch6/1 -> r_NormDwnFilterFac/1
  Switch4/1 -> r_NormUppFilterFac/1
  kmph_VehLgtSpd/1 -> Abs/1
  Compare To Constant1/1 -> Logical Operator/2, Logical Operator2/1
  s_ShftLvrDly/1 -> Compare To Constant2/1
  Compare To Constant2/1 -> Logical Operator/1
  bool_VehStandStillSts/1 -> Logical Operator1/2
  Compare To Constant/1 -> Logical Operator1/1
  bar_BrkPedlP/1 -> Compare To Constant/1
  Abs/1 -> LookupTable (2-D)1/1, LookupTable (2-D)/1
  Logical Operator2/1 -> Switch1/2, Switch2/2
  p_DTR_BrkUpprRateLim_Nmps1/1 -> Switch1/1
  LookupTable (2-D)1/1 -> Switch2/3
  Switch2/1 -> Switch6/3
  p_DTR_BrkUpprRateLim_Nmps4/1 -> Switch2/1
  bool_BrkPedlPsd/1 -> Logical Operator2/2, Switch8/2
  Product/1 -> Switch1/3
  LookupTable (2-D)/1 -> Product/2
  Switch8/1 -> Product/1
  Constant1/1 -> Switch8/3
  Constant/1 -> Switch8/1
  Logical Operator1/1 -> Switch4/2, Switch6/2
  p_DTR_BrkUpprRateLim_Nmps2/1 -> Switch4/1, Switch6/1
  Switch5/1 -> Switch4/3
  Logical Operator/1 -> Switch5/2
  p_DTR_BrkUpprRateLim_Nmps3/1 -> Switch5/1
  Switch1/1 -> Switch5/3
  pct_AccrPedlVal/1 -> Compare To Constant1/1, LookupTable (2-D)1/2, LookupTable (2-D)/2

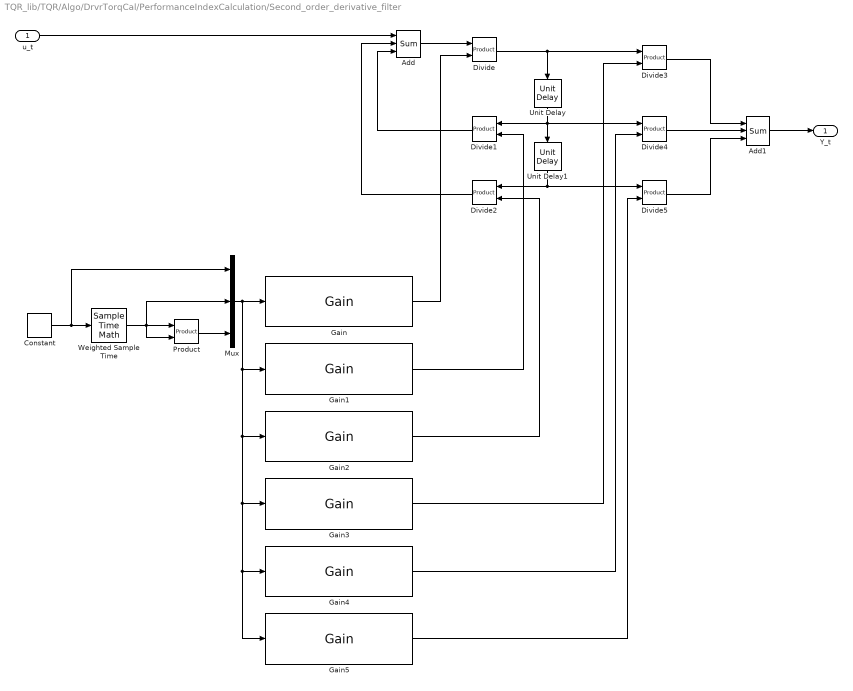
== system TQR_lib/TQR/Algo/DrvrTorqCal/PerformanceIndexCalculation/Second_order_derivative_filter ==
  u_t : Inport
  Add : BaseOperationLib_Browser/Math Operations Changed/Sum  Inputs=+--  OutMin=[]  OutMax=[]  OutDataType=fixdt(1, 16)  OutScaling=2^0
  Add1 : BaseOperationLib_Browser/Math Operations Changed/Sum  Inputs=+++  OutMin=[]  OutMax=[]  OutDataType=fixdt(1, 16)  OutScaling=2^0
  Constant : BaseOperationLib_Browser/Sources&Sinks/Constant  Value=1  OutMin=[]  OutMax=[]  OutDataTypeMode=single  OutDataType=fixdt(1, 16)  ConRadixGroup=Use specified scaling  OutScaling=2^0  OutDataTypeStr=single
  Divide : BaseOperationLib_Browser/Math Operations Changed/Product  Inputs=*/  Multiplication=Element-wise(.*)  OutMin=[]  OutMax=[]  OutDataType=fixdt(1,16,0)  OutScaling=[]
  Divide{1..5} (5 alike) : BaseOperationLib_Browser/Math Operations Changed/Product  Inputs=**  Multiplication=Element-wise(.*)  OutMin=[]  OutMax=[]  OutDataType=fixdt(1,16,0)  OutScaling=[]
  Gain : BaseOperationLib_Browser/Math Operations Changed/Gain  Gain=pTQR_r_PICFilDen1_C  Multiplication=Matrix(K*u)  ParamMin=[]  ParamMax=[]  ParameterDataType=fixdt(1, 16)  ParameterScalingMode=Best Precision: Matrix-wise  ParameterScaling=2^0  OutMin=[]  OutMax=[]  OutDataType=fixdt(1, 16)  OutScaling=2^0
  Gain1 : BaseOperationLib_Browser/Math Operations Changed/Gain  Gain=pTQR_r_PICFilDen2_C  Multiplication=Matrix(K*u)  ParamMin=[]  ParamMax=[]  ParameterDataType=fixdt(1, 16)  ParameterScalingMode=Best Precision: Matrix-wise  ParameterScaling=2^0  OutMin=[]  OutMax=[]  OutDataType=fixdt(1, 16)  OutScaling=2^0
  Gain2 : BaseOperationLib_Browser/Math Operations Changed/Gain  Gain=pTQR_r_PICFilDen3_C  Multiplication=Matrix(K*u)  ParamMin=[]  ParamMax=[]  ParameterDataType=fixdt(1, 16)  ParameterScalingMode=Best Precision: Matrix-wise  ParameterScaling=2^0  OutMin=[]  OutMax=[]  OutDataType=fixdt(1, 16)  OutScaling=2^0
  Gain3 : BaseOperationLib_Browser/Math Operations Changed/Gain  Gain=pTQR_r_PICFilNum1_C  Multiplication=Matrix(K*u)  ParamMin=[]  ParamMax=[]  ParameterDataType=fixdt(1, 16)  ParameterScalingMode=Best Precision: Matrix-wise  ParameterScaling=2^0  OutMin=[]  OutMax=[]  OutDataType=fixdt(1, 16)  OutScaling=2^0
  Gain4 : BaseOperationLib_Browser/Math Operations Changed/Gain  Gain=pTQR_r_PICFilNum2_C  Multiplication=Matrix(K*u)  ParamMin=[]  ParamMax=[]  ParameterDataType=fixdt(1, 16)  ParameterScalingMode=Best Precision: Matrix-wise  ParameterScaling=2^0  OutMin=[]  OutMax=[]  OutDataType=fixdt(1, 16)  OutScaling=2^0
  Gain5 : BaseOperationLib_Browser/Math Operations Changed/Gain  Gain=pTQR_r_PICFilNum3_C  Multiplication=Matrix(K*u)  ParamMin=[]  ParamMax=[]  ParameterDataType=fixdt(1, 16)  ParameterScalingMode=Best Precision: Matrix-wise  ParameterScaling=2^0  OutMin=[]  OutMax=[]  OutDataType=fixdt(1, 16)  OutScaling=2^0
  Mux : Mux  Inputs=3
  Product : BaseOperationLib_Browser/Math Operations Changed/Product  Inputs=2  Multiplication=Element-wise(.*)  OutMin=[]  OutMax=[]  OutDataType=fixdt(1,16,0)  OutScaling=[]  RndMeth=Zero
  Unit Delay : BaseOperationLib_Browser/Discrete Unchanged /Unit Delay  X0=0  SampleTime=-1
  Unit Delay1 : BaseOperationLib_Browser/Discrete Unchanged /Unit Delay  X0=0  SampleTime=-1
  Weighted Sample Time : SampleTimeMath  TsampMathOp=Ts Only
  Y_t : Outport
  wires:
  Gain5/1 -> Divide5/2
  Gain4/1 -> Divide4/2
  Gain3/1 -> Divide3/2
  Gain2/1 -> Divide2/2
  Gain1/1 -> Divide1/2
  Gain/1 -> Divide/2
  Mux/1 -> Gain4/1, Gain5/1, Gain3/1, Gain2/1, Gain1/1, Gain/1
  Product/1 -> Mux/3
  Weighted Sample Time/1 -> Product/2, Mux/2, Product/1
  Constant/1 -> Mux/1, Weighted Sample Time/1
  Add/1 -> Divide/1
  Unit Delay/1 -> Unit Delay1/1, Divide1/1, Divide4/1
  Divide1/1 -> Add/3
  Divide2/1 -> Add/2
  Unit Delay1/1 -> Divide2/1, Divide5/1
  Divide4/1 -> Add1/2
  Divide/1 -> Unit Delay/1, Divide3/1
  Divide5/1 -> Add1/3
  Divide3/1 -> Add1/1
  Add1/1 -> Y_t/1
  u_t/1 -> Add/1

== system TQR_lib/TQR/Algo/DrvrTorqCal/SlpVehLgtSpdTrans/ECrpVehSpdFilter ==
  kmph_VehSpd : Inport
  Abs : BaseOperationLib_Browser/Math Operations Changed/Abs  OutMax=[]  OutDataType=fixdt(1, 16)  OutScaling=2^0  SaturateOnIntegerOverflow=on
  Lookup Table1 : BaseOperationLib_Browser/Lookup Tables Changed/Lookup Table  InputValues=pTQR_kmph_VehSpd_TAB  Table=pTQR_r_VehSpdFilterFac_CUR  LookUpMeth=Interpolation-Use End Values  OutMin=[]  OutMax=[]  OutDataType=fixdt(1, 16)  OutScaling=2^0  OutDataTypeStr=Inherit: Inherit via back propagation  SaturateOnIntegerOverflow=on
      settings: AttributesFormatString=X:%<InputValues>\nTAB:%<Table>
  Unit Delay1 : BaseOperationLib_Browser/Discrete Unchanged /Unit Delay  X0=0  SampleTime=-1
  WerghtingFilter : BaseOperationLib_Browser/Discontinuities Unchanged/WerghtingFilter  SystemSampleTime=-1
  kmph_VehSpdFilter : Outport
  wires:
  kmph_VehSpd/1 -> Abs/1, WerghtingFilter/1
  Unit Delay1/1 -> WerghtingFilter/2
  WerghtingFilter/1 -> Unit Delay1/1, kmph_VehSpdFilter/1
  Lookup Table1/1 -> WerghtingFilter/3
  Abs/1 -> Lookup Table1/1

== system TQR_lib/TQR/Algo/TorqArbitrition/DrivewayAssistTorqArbitrition/ShiftDelayTime ==
  st_ShiftLvrPosn : Inport  PortDimensions=1  OutDataType=fixdt(1, 16)  OutScaling=2^0
  Constant5 : Constant  Value=pTQR_s_SmplCyc_C  OutDataType=Enum: ShiftLvrPosnICTyp  ConRadixGroup=Best Precision: Vector-wise
      mask Display: patch([0 1 1 1 .75], [1 1 0 .75 1], [0 1 0]);
  Discrete-Time Integrator2 : DiscreteIntegrator  IntegratorMethod=Accumulation: Forward Euler  ExternalReset=falling  SampleTime=-1  OutDataType=PDT_s  OutDataTypeStr=Inherit: Inherit via back propagation  LimitOutput=on  UpperSaturationLimit=200  LowerSaturationLimit=0  ICPrevOutput=DiscIntNeverNeededParam  ICPrevScaledInput=DiscIntNeverNeededParam
  Product : BaseOperationLib_Browser/Math Operations Changed/Product  Inputs=2  Multiplication=Element-wise(.*)  OutMin=[]  OutMax=[]  OutDataType=fixdt(1,16,0)  OutScaling=[]  OutDataTypeStr=Inherit: Inherit via back propagation  RndMeth=Zero  SaturateOnIntegerOverflow=on
  Relational Operator1 : RelationalOperator  Operator===  LogicOutDataTypeMode=boolean  OutDataTypeStr=boolean
  Unit Delay3 : UnitDelay  SampleTime=-1
  s_ShftLvrDly : Outport  PortDimensions=1  OutDataType=fixdt(1, 16)  OutScaling=2^0
  wires:
  Product/1 -> s_ShftLvrDly/1
  Constant5/1 -> Product/2
  Discrete-Time Integrator2/1 -> Product/1
  Unit Delay3/1 -> Relational Operator1/2  "st_ActLvrLast"
  Relational Operator1/1 -> Discrete-Time Integrator2/2, Discrete-Time Integrator2/1
  st_ShiftLvrPosn/1 -> Relational Operator1/1, Unit Delay3/1

== system TQR_lib/TQR/Algo/TorqArbitrition/DrivewayAssistTorqArbitrition/Vehicle_StandStill_Status ==
  rpm_MotCtlrActRev : Inport  OutDataType=fixdt(1, 16)  OutScaling=2^0
  Abs : BaseOperationLib_Browser/Math Operations Changed/Abs  OutMax=[]  OutDataType=fixdt(1, 16)  OutScaling=2^0  SaturateOnIntegerOverflow=on
  Chart_VehStandStill : Stateflow chart  TreatAsAtomicUnit=on
  Constant3 : BaseOperationLib_Browser/Sources&Sinks/Constant  Value=pTQR_rpm_VehStdStlSpdThrsh_C  OutMin=[]  OutMax=[]  OutDataTypeMode=single  OutDataType=fixdt(1, 16)  ConRadixGroup=Use specified scaling  OutScaling=2^0  OutDataTypeStr=single
  Constant5 : BaseOperationLib_Browser/Sources&Sinks/Constant  Value=pTQR_rpm_VehMoveSpdThrsh_C  OutMin=[]  OutMax=[]  OutDataTypeMode=single  OutDataType=fixdt(1, 16)  ConRadixGroup=Use specified scaling  OutScaling=2^0  OutDataTypeStr=single
  Constant8 : BaseOperationLib_Browser/Sources&Sinks/Constant  Value=pTQR_s_VehStdStlDly_C  OutMin=[]  OutMax=[]  OutDataTypeMode=single  OutDataType=fixdt(1, 16)  ConRadixGroup=Use specified scaling  OutScaling=2^0  OutDataTypeStr=single
  VehStandStillSts : Outport
  wires:
  Abs/1 -> Chart_VehStandStill/1(rpm_MotCtlrActRev)
  Chart_VehStandStill/1(bool_VehStandStillSt) -> VehStandStillSts/1
  rpm_MotCtlrActRev/1 -> Abs/1
  Constant3/1 -> Chart_VehStandStill/2(rpm_VehStdStlSpdThrsh)
  Constant5/1 -> Chart_VehStandStill/3(rpm_VehMoveSpdThrsh)
  Constant8/1 -> Chart_VehStandStill/4(s_VehStdStlDly)

== system TQR_lib/TQR/Algo/TorqueLimit/no_recuperation/GetBit1 ==
  In1 : Inport
  Bitwise Operator : simulink/Logic and Bit Operations/Bitwise Operator  logicop=AND  UseBitMask=on  BitMask=eval(maska)  BitMaskRealWorld=Stored Integer
  Compare To Zero : simulink/Logic and Bit Operations/Compare To Zero  SystemSampleTime=-1  relop=>  LogicOutDataTypeMode=uint8
  Out1 : Outport
  wires:
  Compare To Zero/1 -> Out1/1
  Bitwise Operator/1 -> Compare To Zero/1
  In1/1 -> Bitwise Operator/1

== system TQR_lib/TQR/Algo/TorqueLimit/torque_reduction/GetBit2 ==
  In1 : Inport
  Bitwise Operator : simulink/Logic and Bit Operations/Bitwise Operator  logicop=AND  UseBitMask=on  BitMask=eval(maska)  BitMaskRealWorld=Stored Integer
  Compare To Zero : simulink/Logic and Bit Operations/Compare To Zero  SystemSampleTime=-1  relop=>  LogicOutDataTypeMode=uint8
  Out1 : Outport
  wires:
  In1/1 -> Bitwise Operator/1
  Bitwise Operator/1 -> Compare To Zero/1
  Compare To Zero/1 -> Out1/1

== system TQR_lib/TQR/Algo/TorqueLimit/velocity_reduction/GetBit1 ==
  In1 : Inport
  Bitwise Operator : simulink/Logic and Bit Operations/Bitwise Operator  logicop=AND  UseBitMask=on  BitMask=eval(maska)  BitMaskRealWorld=Stored Integer
  Compare To Zero : simulink/Logic and Bit Operations/Compare To Zero  SystemSampleTime=-1  relop=>  LogicOutDataTypeMode=uint8
  Out1 : Outport
  wires:
  Compare To Zero/1 -> Out1/1
  Bitwise Operator/1 -> Compare To Zero/1
  In1/1 -> Bitwise Operator/1

== system TQR_lib/TQR/Algo/TorqueLimit/velocity_reduction/GetBit2 ==
  In1 : Inport
  Bitwise Operator : simulink/Logic and Bit Operations/Bitwise Operator  logicop=AND  UseBitMask=on  BitMask=eval(maska)  BitMaskRealWorld=Stored Integer
  Compare To Zero : simulink/Logic and Bit Operations/Compare To Zero  SystemSampleTime=-1  relop=>  LogicOutDataTypeMode=uint8
  Out1 : Outport
  wires:
  In1/1 -> Bitwise Operator/1
  Bitwise Operator/1 -> Compare To Zero/1
  Compare To Zero/1 -> Out1/1

== stateflow chart TQR/Algo/BrakeOverride/Chart ==
  state Normal
    entry:
    bool_OverrideActive = false;
    bool_TqLimit = false;
  state Override
    state ActiveDealy
    state OverrideActive
      entry:
      bool_OverrideActive = true;
    Override.ActiveDealy -> OverrideActive : [after(pTQR_s_AccPedActDly_C,sec)]
    (default) -> Override.ActiveDealy
  state TqLimit
    state ActiveDealy
      entry:
      bool_TqLimit = true;
      bool_OverrideActive = false;
    (default) -> TqLimit.ActiveDealy
  Normal -> Override : [bool_BrkPedlPsd]
  Override -> Normal [order 1] : [!bool_BrkPedlPsd]
  TqLimit -> Normal : [!bool_BrkPedlPsd]
  Override -> TqLimit [order 2] : [ratio_AccrPedlGrad > pTQR_ratio_BrkOvrAccPedGrdTh_C|| ...
      | pct_AccrPedlVal<=pTQR_pct_AccPedAcvThd_C]
  (default) -> Normal
  data: pct_AccrPedlVal input double; ratio_AccrPedlGrad input double; bool_BrkPedlPsd input double; pTQR_s_AccPedActDly_C parameter double; bool_OverrideActive output boolean; bool_TqLimit output boolean; pTQR_ratio_BrkOvrAccPedGrdTh_C parameter double; pTQR_pct_AccPedAcvThd_C parameter double

== stateflow chart TQR/Algo/TorqArbitrition/DrivewayAssistTorqArbitrition/Vehicle_StandStill_Status/Chart_VehStandStill ==
  state VehStandStill
    en:
    bool_VehStandStillSt = true;
  state VehMove
    en:
    bool_VehStandStillSt = false;
  state VehStandStill_Delay
  (default) -> VehStandStill
  VehStandStill -> VehMove : [rpm_MotCtlrActRev>=rpm_VehMoveSpdThrsh]
  VehStandStill_Delay -> VehStandStill [order 2] : [rpm_MotCtlrActRev<rpm_VehStdStlSpdThrsh&& ...
      | after(s_VehStdStlDly, sec)]
  VehMove -> VehStandStill_Delay : [rpm_MotCtlrActRev<rpm_VehStdStlSpdThrsh]
  VehStandStill_Delay -> VehMove [order 1] : [rpm_MotCtlrActRev>=rpm_VehStdStlSpdThrsh]
  data: rpm_MotCtlrActRev input double; bool_VehStandStillSt output boolean; rpm_VehStdStlSpdThrsh input double; rpm_VehMoveSpdThrsh input double; s_VehStdStlDly input double

== stateflow chart TQR/Algo/ACCIntv/trq_arbitration ==
  state normal
    en:normal;
    du:normal;
  state active
    en:active;
    du:active;
  state deactive_dely
    en:deactive_dely;
    du:deactive_dely;
  (default) -> normal
  normal -> active : [active_flg==true]
  active -> deactive_dely : [active_flg==false]
  deactive_dely -> normal [order 1] : [abs(req_trq-feedback_trq)<=Nm_DelyOutTrq]
  deactive_dely -> active [order 2] : [active_flg==true]
  data: active_flg input double; req_trq input double; feedback_trq input double; Nm_DelyOutTrq input double
  events: normal output FUNCTION_CALL_EVENT; active output FUNCTION_CALL_EVENT; deactive_dely output FUNCTION_CALL_EVENT
